simulink model "BallBeam"  (R2021a)
settings: Solver=FixedStepAuto  StartTime=0.0  StopTime=20  FixedStep=0.001  RelTol=1e-3
undefined symbols (not defined in the file or in its folder): d1, g, J, m
libraries: sm_lib x2, pid_lib x1, robotcorelib x1
settings Model: Creator=fabio  LastModifiedBy=fede
settings SolverCC: AlgebraicLoopSolver=TrustRegion
settings DebuggingCC: SFMachineParentedDataDiag=warning

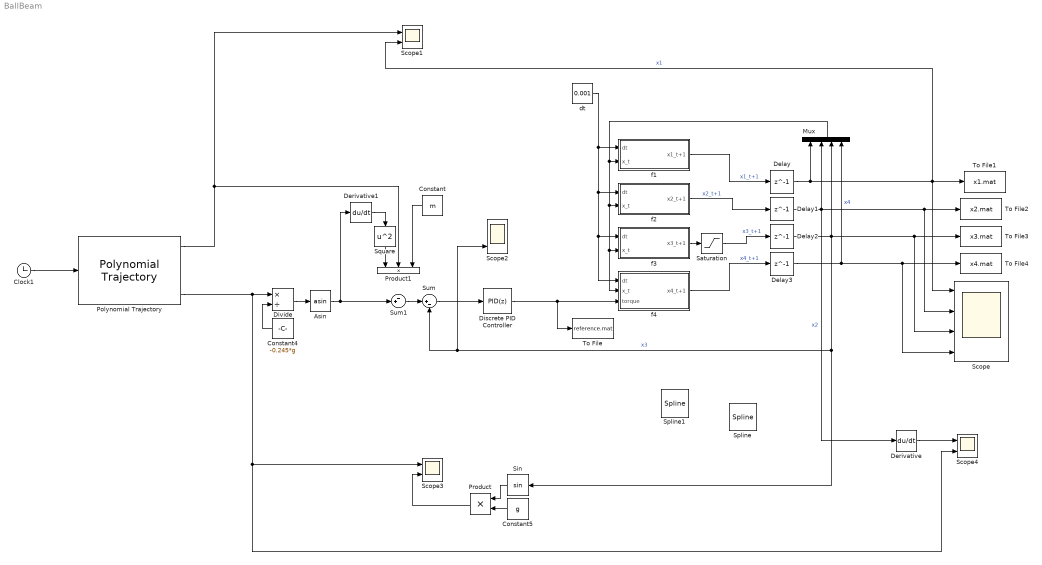
== system BallBeam ==
  Asin : Trigonometry  Operator=asin
  Clock1 : Clock
  Constant : Constant  Value=m
  Constant4 : Constant  Value=-0.245*g
  Constant5 : Constant  Value=g
  Delay : Delay  DelayLength=1  InitialCondition=0  SampleTime=0.001
  Delay1 : Delay  DelayLength=1  SampleTime=0.001
  Delay2 : Delay  DelayLength=1  InitialCondition=0  SampleTime=0.001
  Delay3 : Delay  DelayLength=1  SampleTime=0.001
  Derivative : Derivative
  Derivative1 : Derivative
  Discrete PID Controller : pid_lib/PID Controller  Controller=PID  Form=Parallel  TimeDomain=Discrete-time  UseExternalTs=off  SampleTime=0.001  IntegratorMethod=Forward Euler  FilterMethod=Forward Euler  ControllerParametersSource=internal  P=-3.21632974412931  I=-5.13866455963317  D=-0.330228892717756  UseFilter=on  N=354.523079816962  TunerSelectOption=Transfer Function Based (PID Tuner App)  InitialConditionSource=internal  InitialConditionForIntegrator=0  InitialConditionForFilter=0  DifferentiatorICPrevScaledInput=0  ExternalReset=none  TrackingMode=off  Kt=1  LimitOutput=off  SatLimitsSource=internal  UpperSaturationLimit=inf  LowerSaturationLimit=-inf  LinearizeAsGain=off  AntiWindupMode=none  Kb=1  POutMin=[]  POutMax=[]  IOutMin=[]  IOutMax=[]  DOutMin=[]  DOutMax=[]  NOutMin=[]  NOutMax=[]  SumOutMin=[]  SumOutMax=[]  SaturationOutMin=[]  SaturationOutMax=[]  PParamMin=[]  PParamMax=[]  IParamMin=[]  IParamMax=[]  DParamMin=[]  DParamMax=[]  NParamMin=[]  NParamMax=[]  KbParamMin=[]  KbParamMax=[]  KtParamMin=[]  KtParamMax=[]  KbOutMin=[]  KbOutMax=[]  KtOutMin=[]  KtOutMax=[]  IntegratorOutMin=[]  IntegratorOutMax=[]  FilterOutMin=[]  FilterOutMax=[]  SumI1OutMin=[]  SumI1OutMax=[]  SumI2OutMin=[]  SumI2OutMax=[]  SumI3OutMin=[]  SumI3OutMax=[]  SumI4OutMin=[]  SumI4OutMax=[]  SumDOutMin=[]  SumDOutMax=[]  DifferentiatorOutMin=[]  DifferentiatorOutMax=[]  FilterDiffOutCoefMin=[]  FilterDiffOutCoefMax=[]  ReciprocalOutMin=[]  ReciprocalOutMax=[]  SumDenOutMin=[]  SumDenOutMax=[]  SumNumOutMin=[]  SumNumOutMax=[]  DivideOutMin=[]  DivideOutMax=[]  UdiffTsProdOutMin=[]  UdiffTsProdOutMax=[]  NTsProdOutMin=[]  NTsProdOutMax=[]  UintegralTsProdOutMin=[]  UintegralTsProdOutMax=[]  UngainTsProdOutMin=[]  UngainTsProdOutMax=[]  IntegratorContinuousStateAttributes=''  IntegratorStateMustResolveToSignalObject=off  IntegratorRTWStateStorageClass=Auto  FilterContinuousStateAttributes=''  FilterStateMustResolveToSignalObject=off  FilterRTWStateStorageClass=Auto  ParallelPVariant=InternalParameters  IdealPVariant=Disabled  IVariant=InternalParameters  DVariant=InternalParameters  IntegratorVariant=Discrete  SatVariant=Disabled  AWVariant=Passthrough  PCopyVariant=Disabled  TRVariant=Disabled  FdbkBlocksVariant=Forward  IdealPFdbkVariant=Disabled  SatFdbkVariant=Disabled  DerivativeFilterVariant=ForwardEulerFilter  NVariant=InternalParameters  NCopyVariant=Disabled  FilterICVariant=InternalICsFilter  IntegratorICVariant=InternalICs  ExternalResetVariant=Disabled  TRSumVariant=Passthrough  SumFdbkVariant=Disabled  SumVariant=Sum_PID  TsampFilterVariant=InternalTs  TsampNgainVariant=Passthrough  TsampIntegralVariant=Passthrough  ExternalSaturationOutDataTypeStr=Inherit: Same as second input
  Divide : Product  Inputs=*/
  Mux : Mux
  Polynomial Trajectory : robotcorelib/Polynomial Trajectory  WaypointSource=Internal  Waypoints=p  TimePoints=my_tpts  TimeInterval=[ 0, 1, 2.5, 3 ]  Method=Quintic Polynomial  ParameterSource=Internal  VelocityBoundaryCondition=p_dot  AccelerationBoundaryCondition=p_ddot  SimulateUsing=Interpreted execution
  Product : Product
  Product1 : Product  Inputs=3
  Saturation : Saturate  UpperLimit=pi/4  LowerLimit=-pi/4
  Scope : Scope  NumInputPorts=4
  Scope1 : Scope  NumInputPorts=2
  Scope2 : Scope  NumInputPorts=3
  Scope3 : Scope  NumInputPorts=2
  Scope4 : Scope  NumInputPorts=2
  Sin : Trigonometry
  Spline : sm_lib/Curves and Surfaces/Spline  GraphicAmbientColor=[0.15 0.15 0.15 1.0]  GraphicDiffuseColor=[0.0 0.0 0.0]  DataPoints=[6 -2 9;-6 5 -4;-6 -7 9;6 0 -4;-3 6 9;-3 -8 -4]  DataPointsUnits=m  GraphicEmissiveColor=[0.0 0.0 0.0 1.0]  EndConditionType=Closed  MarkerShape=Sphere  MarkerSize=10  GraphicType=FromGeometry  GraphicOpacity=1.0  GraphicShininess=75  GraphicSpecularColor=[0.5 0.5 0.5 1.0]  GraphicVisPropType=SimpleVisualProperties
  Spline1 : sm_lib/Curves and Surfaces/Spline  GraphicAmbientColor=[0.15 0.15 0.15 1.0]  GraphicDiffuseColor=[0.0 0.0 0.0]  DataPoints=[6 -2 9;-6 5 -4;-6 -7 9;6 0 -4;-3 6 9;-3 -8 -4]  DataPointsUnits=m  GraphicEmissiveColor=[0.0 0.0 0.0 1.0]  EndConditionType=Closed  MarkerShape=Sphere  MarkerSize=10  GraphicType=FromGeometry  GraphicOpacity=1.0  GraphicShininess=75  GraphicSpecularColor=[0.5 0.5 0.5 1.0]  GraphicVisPropType=SimpleVisualProperties
  Square : Math  Operator=square  SaturateOnIntegerOverflow=on
  Sum : Sum  Inputs=|+-
  Sum1 : Sum  Inputs=-+|
  To File : ToFile  Filename=reference.mat  MatrixName=torque
  To File1 : ToFile  Filename=x1.mat  MatrixName=x1
  To File2 : ToFile  Filename=x2.mat  MatrixName=x2
  To File3 : ToFile  Filename=x3.mat  MatrixName=x3
  To File4 : ToFile  Filename=x4.mat  MatrixName=x4
  dt : Constant  Value=0.001
  f1 : Subsystem
  f2 : Subsystem
  f3 : Subsystem
  f4 : Subsystem
  wires:
  f1/1(x1_t+1) -> Delay/1  "x1_t+1"
  f2/1(x2_t+1) -> Delay1/1  "x2_t+1"
  f4/1(x4_t+1) -> Delay3/1  "x4_t+1"
  Delay/1 -> Scope1/2, Scope/1, To File1/1, Mux/1  "x1"
  dt/1 -> f4/1(dt), f3/1(dt), f2/1(dt), f1/1(dt)
  Delay1/1 -> Scope/2, To File2/1, Derivative/1, Mux/2  "x2"
  Delay3/1 -> Scope/4, To File4/1, Mux/4  "x4"
  Mux/1 -> f3/2(x_t), f4/2(x_t), f2/2(x_t), f1/2(x_t)
  Delay2/1 -> Scope/3, To File3/1, Mux/3, Sin/1, Scope2/3, Sum/2  "x3"
  f3/1(x3_t+1) -> Saturation/1
  Saturation/1 -> Delay2/1  "x3_t+1"
  Polynomial Trajectory/3 -> Scope3/1, Scope4/2, Divide/1
  Constant4/1 -> Divide/2
  Sum/1 -> Discrete PID Controller/1
  Discrete PID Controller/1 -> To File/1, f4/3(torque)
  Divide/1 -> Asin/1
  Polynomial Trajectory/1 -> Scope1/1, Product1/2
  Constant5/1 -> Product/2
  Sin/1 -> Product/1
  Product/1 -> Scope3/2
  Clock1/1 -> Polynomial Trajectory/1
  Derivative/1 -> Scope4/1
  Asin/1 -> Derivative1/1, Sum1/2
  Sum1/1 -> Sum/1
  Square/1 -> Product1/1
  Constant/1 -> Product1/3
  Derivative1/1 -> Square/1

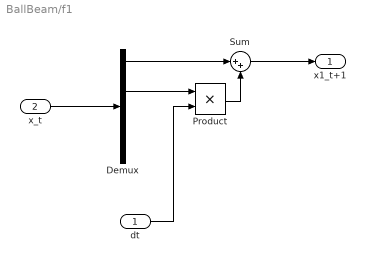
== system BallBeam/f1 ==
  dt : Inport
  x_t : Inport  Port=2
  Demux : Demux
  Product : Product
  Sum : Sum  Inputs=|++
  x1_t+1 : Outport
  wires:
  x_t/1 -> Demux/1
  Demux/1 -> Sum/1
  Demux/2 -> Product/1
  dt/1 -> Product/2
  Product/1 -> Sum/2
  Sum/1 -> x1_t+1/1

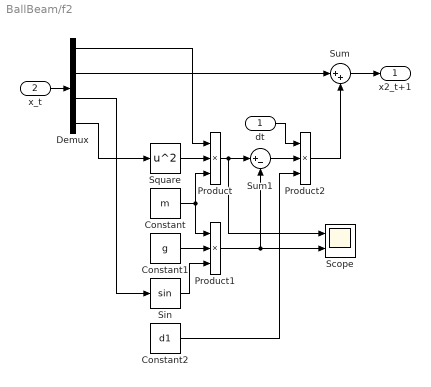
== system BallBeam/f2 ==
  dt : Inport
  x_t : Inport  Port=2
  Constant : Constant  Value=m
  Constant1 : Constant  Value=g
  Constant2 : Constant  Value=d1
  Demux : Demux
  Product : Product  Inputs=3
  Product1 : Product  Inputs=3
  Product2 : Product  Inputs=3
  Scope : Scope  NumInputPorts=2
  Sin : Trigonometry
  Square : Math  Operator=square  SaturateOnIntegerOverflow=on
  Sum : Sum  Inputs=|++
  Sum1 : Sum  Inputs=|+-
  x2_t+1 : Outport
  wires:
  x_t/1 -> Demux/1
  Sum/1 -> x2_t+1/1
  Square/1 -> Product/2
  Demux/4 -> Square/1
  Constant/1 -> Product/3, Product1/1
  Product/1 -> Scope/1, Sum1/1
  Demux/3 -> Sin/1
  Sin/1 -> Product1/3
  Constant1/1 -> Product1/2
  Product1/1 -> Scope/2, Sum1/2
  Sum1/1 -> Product2/2
  dt/1 -> Product2/1
  Product2/1 -> Sum/2
  Constant2/1 -> Product2/3
  Demux/2 -> Sum/1
  Demux/1 -> Product/1

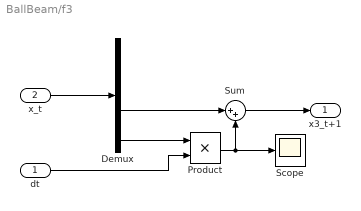
== system BallBeam/f3 ==
  dt : Inport
  x_t : Inport  Port=2
  Demux : Demux
  Product : Product
  Scope : Scope
  Sum : Sum  Inputs=|++
  x3_t+1 : Outport
  wires:
  x_t/1 -> Demux/1
  Product/1 -> Scope/1, Sum/2
  dt/1 -> Product/2
  Demux/3 -> Sum/1
  Sum/1 -> x3_t+1/1
  Demux/4 -> Product/1

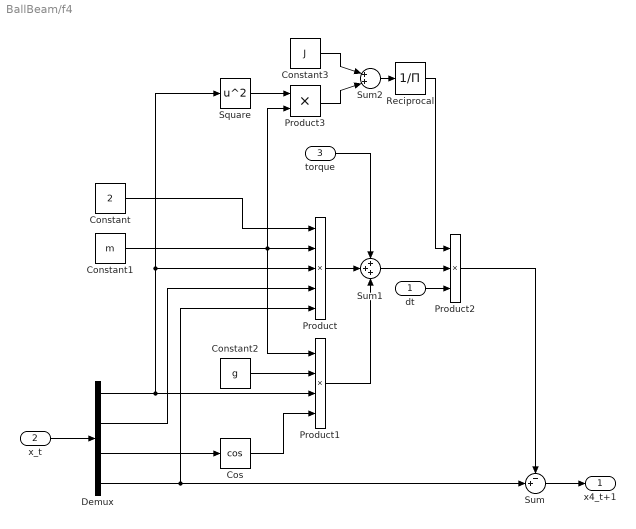
== system BallBeam/f4 ==
  dt : Inport
  x_t : Inport  Port=2
  torque : Inport  Port=3
  Constant : Constant  Value=2
  Constant1 : Constant  Value=m
  Constant2 : Constant  Value=g
  Constant3 : Constant  Value=J
  Cos : Trigonometry  Operator=cos
  Demux : Demux
  Product : Product  Inputs=5
  Product1 : Product  Inputs=4
  Product2 : Product  Inputs=3
  Product3 : Product
  Reciprocal : Product  Inputs=/
  Square : Math  Operator=square  SaturateOnIntegerOverflow=on
  Sum : Sum  Inputs=-+|
  Sum1 : Sum  Inputs=+++
  Sum2 : Sum  Inputs=|++|
  x4_t+1 : Outport
  wires:
  x_t/1 -> Demux/1
  Sum/1 -> x4_t+1/1
  Demux/4 -> Product/5, Sum/2
  Constant/1 -> Product/1
  Constant1/1 -> Product1/1, Product3/2, Product/2
  Demux/1 -> Square/1, Product/3, Product1/3
  Demux/2 -> Product/4
  Constant2/1 -> Product1/2
  Demux/3 -> Cos/1
  Cos/1 -> Product1/4
  Product/1 -> Sum1/2
  torque/1 -> Sum1/1
  Product1/1 -> Sum1/3
  Sum1/1 -> Product2/2
  dt/1 -> Product2/3
  Product2/1 -> Sum/1
  Square/1 -> Product3/1
  Product3/1 -> Sum2/2
  Constant3/1 -> Sum2/1
  Sum2/1 -> Reciprocal/1
  Reciprocal/1 -> Product2/1
